simulink model "biquad_test_v4_old"  (R2024b)
settings: Solver=FixedStepDiscrete  StartTime=0.0  StopTime=T  RelTol=1e-12
values from neighbouring files (symbols this model uses):
  a1 = sos_fix(1,5)    [Biquad_Test_Filter_v3.m]    (also in Biquad_Test_Filter_v4.m)
  a2 = sos_fix(1,6)    [Biquad_Test_Filter_v3.m]    (also in Biquad_Test_Filter_v4.m)
  b0 = sos_fix(1,1)    [Biquad_Test_Filter_v3.m]    (also in Biquad_Test_Filter_v4.m)
  b1 = sos_fix(1,2)    [Biquad_Test_Filter_v3.m]    (also in Biquad_Test_Filter_v4.m)
  b2 = sos_fix(1,3)    [Biquad_Test_Filter_v3.m]    (also in Biquad_Test_Filter_v4.m)
  Fs = 44100    [Biquad_Test_Filter_v3.m]    (also in Biquad_Test_Filter_v4.m; Biquad_Test_Filter_v4_test.m; Biquad_Test_Filter_v5_test.m = 48000; Biquad_Test_Filter_v6_test.m = 48000)
libraries: dspsrcs4 x1
settings Model: DataTypeOverride=Off  Creator=korvo  LastModifiedBy=korvo
settings OptimizationCC: BlockReduction=off  ConditionallyExecuteInputs=off  DefaultParameterBehavior=Inlined  InheritOutputTypeSmallerThanSingle=on
settings DebuggingCC: AlgebraicLoopMsg=error  ArtificialAlgebraicLoopMsg=error  SingleTaskRateTransMsg=error  UnconnectedInputMsg=warning  UnconnectedOutputMsg=warning  UnconnectedLineMsg=warning
settings HardwareCC: ProdBitPerPointer=32  ProdBitPerSizeT=32  ProdBitPerPtrDiffT=32  ProdLargestAtomicFloat=None  ProdIntDivRoundTo=Undefined  ProdEndianess=Unspecified  ProdWordSize=32  ProdHWDeviceType=ASIC/FPGA->ASIC/FPGA  TargetBitPerPointer=64  TargetBitPerSizeT=64  TargetBitPerPtrDiffT=64  TargetLongLongMode=on  TargetIntDivRoundTo=Zero  TargetEndianess=LittleEndian  TargetWordSize=64  TargetHWDeviceType=Custom Processor->MATLAB Host Computer  ProdEqTarget=off

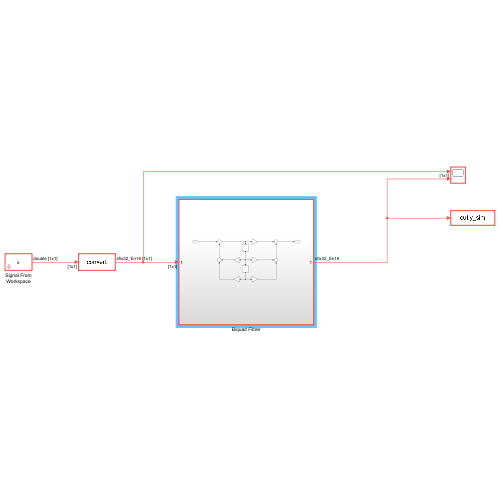
[thumbnail: Simulink's stored preview of the top-level diagram]
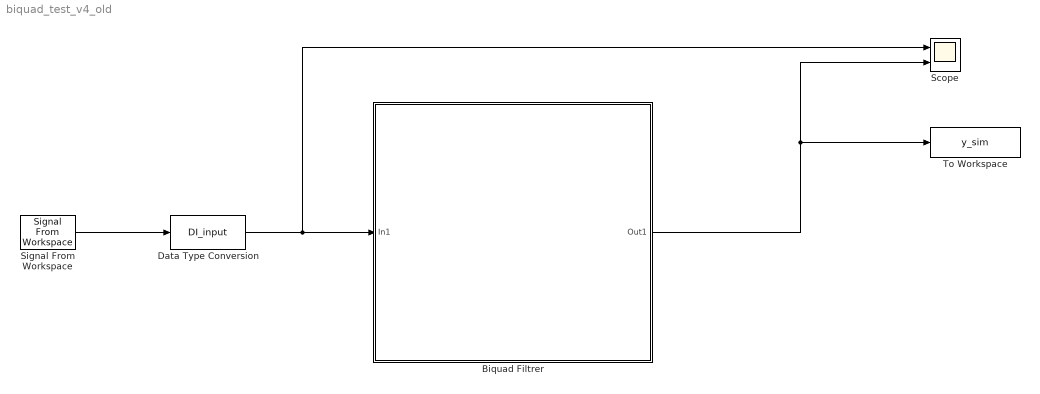
== system biquad_test_v4_old ==
  Biquad Filtrer : Subsystem
  Data Type Conversion : DataTypeConversion  OutDataTypeStr=DI_input  SaturateOnIntegerOverflow=off  RndMeth=Floor
  Scope : Scope  NumInputPorts=2
  Signal From Workspace : dspsrcs4/Signal From Workspace  X=x  Ts=1/Fs  nsamps=1  OutputAfterFinalValue=Setting to zero  ignoreOrWarnInputAndFrameLengths=off  OutputFrames=off
  To Workspace : ToWorkspace  VariableName=y_sim  SampleTime=-1
  wires:
  Signal From Workspace/1 -> Data Type Conversion/1
  Data Type Conversion/1 -> Scope/1, Biquad Filtrer/1(In1)
  Biquad Filtrer/1(Out1) -> Scope/2, To Workspace/1

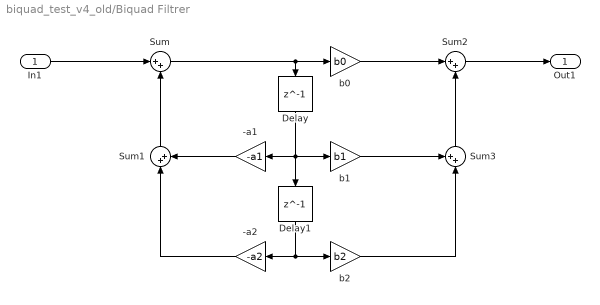
== system biquad_test_v4_old/Biquad Filtrer ==
  In1 : Inport
  -a1 : Gain  Gain=-a1  OutDataTypeStr=DI_input
  -a2 : Gain  Gain=-a2  OutDataTypeStr=DI_input
  Delay : Delay  DelayLength=1
  Delay1 : Delay  DelayLength=1
  Sum : Sum  Inputs=|++  OutDataTypeStr=DI_input  SaturateOnIntegerOverflow=on
  Sum1 : Sum  Inputs=|++  OutDataTypeStr=DI_input  SaturateOnIntegerOverflow=on
  Sum2 : Sum  Inputs=|++  OutDataTypeStr=DI_input  SaturateOnIntegerOverflow=on
  Sum3 : Sum  Inputs=++|  OutDataTypeStr=DI_input  SaturateOnIntegerOverflow=on
  b0 : Gain  Gain=b0  OutDataTypeStr=DI_input
  b1 : Gain  Gain=b1  OutDataTypeStr=DI_input
  b2 : Gain  Gain=b2  OutDataTypeStr=DI_input
  Out1 : Outport
  wires:
  Delay1/1 -> b2/1, -a2/1
  b0/1 -> Sum2/1
  -a1/1 -> Sum1/2
  Sum1/1 -> Sum/2
  In1/1 -> Sum/1
  -a2/1 -> Sum1/1
  Sum/1 -> Delay/1, b0/1
  Sum3/1 -> Sum2/2
  b1/1 -> Sum3/1
  b2/1 -> Sum3/2
  Sum2/1 -> Out1/1
  Delay/1 -> Delay1/1, b1/1, -a1/1
